simulink model "HYDROPOWERPLANTSTIMULATION0x2820x29"  (R2023a)
settings: Solver=VariableStepAuto  StartTime=0.0  StopTime=10  RelTol=1e-3
undefined symbols (not defined in the file): D1, Delta
libraries: spsGroundLib x2, spsThreePhaseParallelRLCLoadLib x2, spsVoltageMeasurementLib x2, spsExcitationSystemLib x1, spsHydraulicTurbineandGovernorLib x1, spsSynchronousMachinepuFundamentalLib x1, spsThreePhaseTransformerTwoWindingsLib x1, spsThreePhaseSourceLib x1, spspowerguiLib x1
settings Model: Creator=DELL  LastModifiedBy=Smile
settings SolverCC: AlgebraicLoopSolver=TrustRegion
settings DebuggingCC: UnconnectedInputMsg=warning  UnconnectedOutputMsg=warning  UnconnectedLineMsg=warning
settings ModelReferenceCC: EnableRefExpFcnMdlSchedulingChecks=on
settings RTWCC: DLArmComputeVersion=19.05

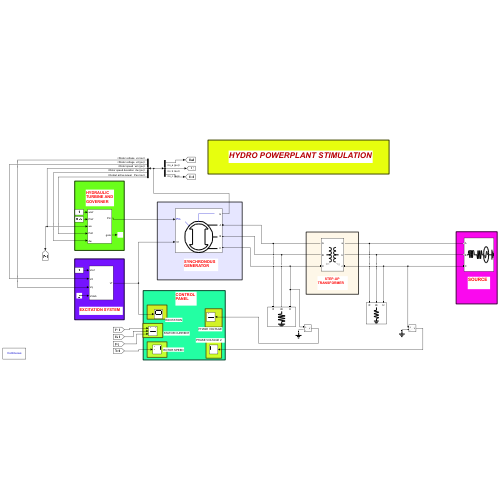
[thumbnail: Simulink's stored preview of the top-level diagram]
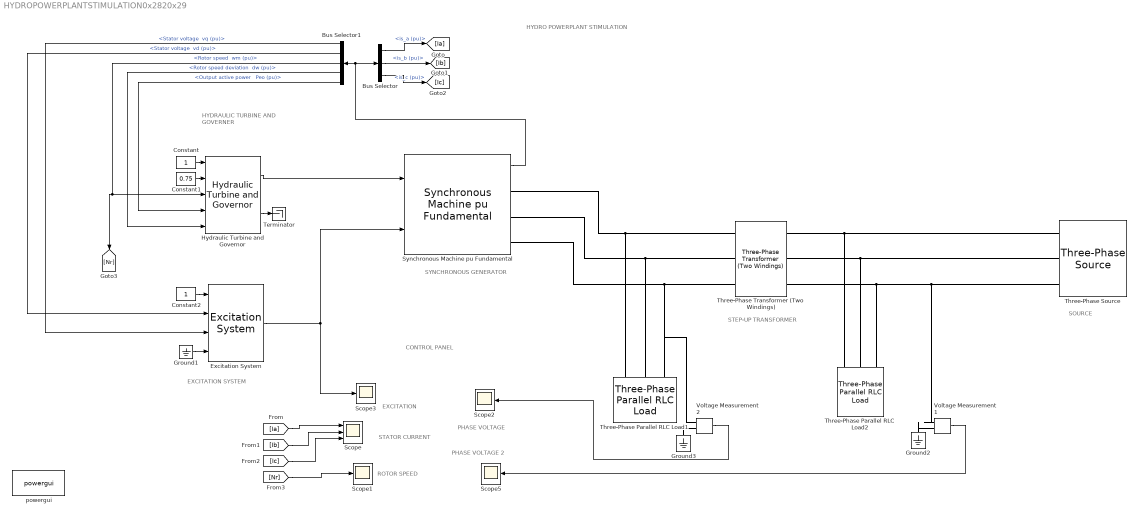
== system HYDROPOWERPLANTSTIMULATION0x2820x29 ==
  note: PHASE VOLTAGE 2
  note: PHASE VOLTAGE
  note: EXCITATION
  note: STATOR CURRENT
  note: ROTOR SPEED
  note: HYDRO POWERPLANT STIMULATION
  note: CONTROL PANEL
  note: EXCITATION SYSTEM
  note: HYDRAULIC TURBINE AND GOVERNER
  note: SOURCE
  note: STEP-UP TRANSFORMER
  note: SYNCHRONOUS GENERATOR
  Bus Selector : BusSelector  OutputSignals=Stator current.is_a (pu),Stator current.is_b (pu),Stator current.is_c (pu)
  Bus Selector1 : BusSelector  OutputSignals="dq0 components.Stator voltage  vq (pu),dq0 components.Stator voltage  vd (pu),Mechanical.Rotor speed  wm (pu),Mechanical.Rotor speed deviation  dw (pu),Output active power   Peo (pu)"
  Constant : Constant
  Constant1 : Constant  Value=0.75
  Constant2 : Constant
  Excitation System : spsExcitationSystemLib/Excitation System  tr=20e-3  reg=[ 300, 0.001 ]  exc=[ 1, 0 ]  tgr=[ 0, 0 ]  damp=[ 0.001, 0.1 ]  sat=[ 0, 0 ]  lim=[ -11.5, 11.5, 0 ]  v0="[1.0  1.28]"
  Ground1 : Ground
  Ground2 : spsGroundLib/Ground  LConnTagsString=a
  Ground3 : spsGroundLib/Ground  LConnTagsString=a
  Hydraulic Turbine and Governor : spsHydraulicTurbineandGovernorLib/Hydraulic Turbine and Governor  sm="[ 10/3  0.07 ]"  gate="[  0.01  0.97518  -0.1  0.1 ]"  reg="[  0.05  1.163  0.105  0  0.01  ]"  hyd="[  0  2.67  ]"  dref=0  po=0.7516
  Scope : Scope  NumInputPorts=3
  Scope{1..3,5} (4 alike) : Scope
  Synchronous Machine pu Fundamental : spsSynchronousMachinepuFundamentalLib/Synchronous Machine pu Fundamental  PresetModel=No  MechanicalLoad=Mechanical power Pm  ShowDetailedParameters=on  RotorType=Salient-pole  Units=per unit fundamental parameters  MeasurementBus=off  NominalParameters="[ 200E6  13800   60]"  Stator="[ 2.85E-03  0.114  1.19  0.36 ]"  Field="[ 5.79E-04  0.114]"  Dampers2=[0.0652, 0.5134, 0.0287, 0.2553, 7.765e-3, 0.9167 ]  Dampers1="[ 1.17E-02  0.182  1.97E-02  0.384 ]"  Mechanical=[ 3.7 0 20]  PolePairs=20  InitialConditions="[ 0  0  0  0  0  0  0  0  1 ]"  SetSaturation=off  Saturation=[0.6404,0.7127,0.8441,0.9214,0.9956,1.082,1.19,1.316,1.457;0.7,0.7698,0.8872,0.9466,0.9969,1.046,1.1,1.151,1.201]  LoadFlowParameters=[1,0,0,0,0]  TsPowergui=0  TsBlock=-1  IterativeModel=Trapezoidal non iterative  IterativeDiscreteModel=Trapezoidal non iterative  BusType=PV  Pref=0  Qref=0  Qmin=-inf  Qmax=inf  PLF=0  QLF=0
  Terminator : Terminator
  Three-Phase Parallel RLC Load1 : spsThreePhaseParallelRLCLoadLib/Three-Phase Parallel RLC Load  LConnTagsString=A|B|C  Configuration=Y (grounded)  NominalVoltage=13800  Vabc=[1e3 1e3 1e3]  Vabcp=[1e3 1e3 1e3]  NominalFrequency=60  UnbalancedPower=off  ActivePower=5e6  InductivePower=0  CapacitivePower=0  Pabc=[10e3 9e3 11e3]  QLabc=[100 90 110]  QCabc=[100 90 110]  Pabcp=[10e3 9e3 11e3]  QLabcp=[100 90 110]  QCabcp=[100 90 110]  Measurements=None  LoadType=constant Z
  Three-Phase Parallel RLC Load2 : spsThreePhaseParallelRLCLoadLib/Three-Phase Parallel RLC Load  LConnTagsString=A|B|C  Configuration=Y (grounded)  NominalVoltage=210e3  Vabc=[1e3 1e3 1e3]  Vabcp=[1e3 1e3 1e3]  NominalFrequency=60  UnbalancedPower=off  ActivePower=10e6  InductivePower=0  CapacitivePower=0  Pabc=[10e3 9e3 11e3]  QLabc=[100 90 110]  QCabc=[100 90 110]  Pabcp=[10e3 9e3 11e3]  QLabcp=[100 90 110]  QCabcp=[100 90 110]  Measurements=None  LoadType=constant Z
  Three-Phase Transformer (Two Windings) : spsThreePhaseTransformerTwoWindingsLib/Three-Phase Transformer (Two Windings)  Winding1Connection=Delta (D1)  Winding2Connection=Yg  CoreType=Three single-phase transformers  SetSaturation=off  Hysteresis=off  DataFile='hysteresis'  SetInitialFlux=off  Measurements=None  UNITS=pu  NominalPower=[ 210e6 , 60 ]  Winding1=[ 13.8e3 , 0.002 , 0.08 ]  Winding2=[ 230e3 , 0.002 , 0.08 ]  Rm=500  Lm=500  L0=0.5  Saturation=[ 0,0 ; 0.0024,1.2 ; 1.0,1.52 ]  InitialFluxes=[ 0.8 , -0.8 , 0.7 ]  BreakLoop=off  DiscreteSolver=Trapezoidal iterative  DataType=off  TransfoNumber=1
  Three-Phase Source : spsThreePhaseSourceLib/Three-Phase Source  InternalConnection=Yg  VoltagePhases=off  Voltage=210e3  PhaseAngle=0  Voltage_phases=[25e3 25e3 25e3]/sqrt(3)  PhaseAngles_phases=[0 -120 +120]  Frequency=60  NonIdealSource=on  SpecifyImpedance=on  Resistance=0.8929  Inductance=16.58e-3  ShortCircuitLevel=10000e6  BaseVoltage=210e3  XRratio=10  BusType=swing  Pref=10e3  Qref=0  Prefabc=[10e3, 10e3, 10e3]  Qrefabc=[0, 0, 0]  Qmin=-inf  Qmax=inf
  Voltage Measurement1 : spsVoltageMeasurementLib/Voltage Measurement  PhasorSimulation=off  OutputType=Complex  PSBequivalent=0
  Voltage Measurement2 : spsVoltageMeasurementLib/Voltage Measurement  PhasorSimulation=off  OutputType=Complex  PSBequivalent=0
  powergui : spspowerguiLib/powergui  Priority=1  SimulationMode=Continuous  SampleTime=50e-6  frequency=60  Iterations=50  frequencyindice=60  Pbase=100e6  ErrMax=1e-4  UnitsV=kV  UnitsW=MW  buscounter=0  FunctionMessages=off  echomessages=off  EnableUseOfTLC=off  CurrentSourceSwitches=off  DisableSnubberDevices=off  DisableRonSwitches=off  DisableVfSwitches=off  DisplayEquations=off  AutomaticDiscreteSolvers=off  SolverType=Tustin/Backward Euler (TBE)  Interpol=off  ExternalGateDelay=off  methode=off  Ts=100  x0status=blocks  SPID=on  SwTol=0  HookPort=off  NonlinearTolerance=1e-4  nMaxIteration=100  ContinueOnMaxIteration=off  RestoreLinks=warning  ResistiveCurrentMeasurement=off  Frange=[0:2:500]  Ylog=off  Xlog=on  ShowGrid=off  save=off  variable=ZData  structure=0  ZoomFFT=off  StartTime=0.0  cycles=1  DisplayStyle=1  fundamental=60  FreqAxis=off  MaxFrequency=1000  frequencyindicesteady=1  RmsSteady=1  display=off
  wires:
  Excitation System/1 -> Synchronous Machine pu Fundamental/2, Scope3/1
  Ground1/1 -> Excitation System/4
  Synchronous Machine pu Fundamental/1 -> Bus Selector/1, Bus Selector1/1
  Bus Selector1/3 -> Hydraulic Turbine and Governor/3, [Nr]  "<Rotor speed  wm (pu)>"
  Constant/1 -> Hydraulic Turbine and Governor/1
  Constant1/1 -> Hydraulic Turbine and Governor/2
  Bus Selector1/4 -> Hydraulic Turbine and Governor/5  "<Rotor speed deviation  dw (pu)>"
  Bus Selector1/5 -> Hydraulic Turbine and Governor/4  "<Output active power   Peo (pu)>"
  Hydraulic Turbine and Governor/2 -> Terminator/1
  Bus Selector1/1 -> Excitation System/3  "<Stator voltage  vq (pu)>"
  Bus Selector1/2 -> Excitation System/2  "<Stator voltage  vd (pu)>"
  Voltage Measurement1/1 -> Scope5/1
  Constant2/1 -> Excitation System/1
  Hydraulic Turbine and Governor/1 -> Synchronous Machine pu Fundamental/1
  Voltage Measurement2/1 -> Scope2/1
  Bus Selector/1 -> [Ia]  "<is_a (pu)>"
  [Ia] -> Scope/1
  Bus Selector/2 -> [Ib]  "<is_b (pu)>"
  [Ib] -> Scope/2
  [Ic] -> Scope/3
  Bus Selector/3 -> [Ic]  "<is_c (pu)>"
  [Nr] -> Scope1/1
  connections:
  Synchronous Machine pu Fundamental/RConn1 -- Three-Phase Parallel RLC Load1/LConn1 -- Three-Phase Transformer (Two Windings)/LConn1
  Synchronous Machine pu Fundamental/RConn2 -- Three-Phase Parallel RLC Load1/LConn2 -- Three-Phase Transformer (Two Windings)/LConn2
  Synchronous Machine pu Fundamental/RConn3 -- Voltage Measurement2/LConn1 -- Three-Phase Parallel RLC Load1/LConn3 -- Three-Phase Transformer (Two Windings)/LConn3
  Three-Phase Transformer (Two Windings)/RConn1 -- Three-Phase Parallel RLC Load2/LConn1 -- Three-Phase Source/RConn1
  Three-Phase Transformer (Two Windings)/RConn2 -- Three-Phase Parallel RLC Load2/LConn2 -- Three-Phase Source/RConn2
  Three-Phase Transformer (Two Windings)/RConn3 -- Voltage Measurement1/LConn1 -- Three-Phase Source/RConn3 -- Three-Phase Parallel RLC Load2/LConn3
  Ground2/LConn1 -- Voltage Measurement1/LConn2
  Voltage Measurement2/LConn2 -- Ground3/LConn1
